simulink model "LabB_PIDOverRobot"  (R2020b)
settings: Solver=FixedStepDiscrete  StartTime=0.0  StopTime=inf  FixedStep=fSamplingPeriod  RelTol=1e-3  EnableMultiTasking=on
values from neighbouring files (symbols this model uses):
  acc_LSB_per_g = 16384    [GyroAccScaling.mat]
  acc_y_offset = 651.5    [OffsetData.mat]
  acc_z_offset = 170.75    [OffsetData.mat]
  fSamplingPeriod = 0.005    [LabB_ControllerOverSimulator_Discrete_Parameters.m]    (also in LabB_ControllerOverSimulator_Discrete_Parameters_conflict_copy_LAPTOP-FOGVCHE7_2020_11_15.m; LabB_ObserverAndControllerOverSimulator_Discrete_Parameters.m; LabC_6_3.m = 0.2; LabC_6_4.m = 0.067)
  fWheelRadius = 0.0216    [LoadRobotParameters.m]
  gyro_LSB_per_deg = 131    [GyroAccScaling.mat]
  gyro_x_offset = -193.125    [OffsetData.mat]
  iNumberOfEncoderSteps = 720    [LoadRobotParameters.m]
  kD = -0.87072    [LabB_ObserverAndControllerOverSimulator_Discrete_Parameters.m]    (also in LabB_ObserverOverSimulator_Continuous_Parameters.m; LabB_ObserverOverSimulator_Discrete_Parameters.m; LabC_6_6.m = 28.69)
  kI = -13776.6318    [LabB_ObserverAndControllerOverSimulator_Discrete_Parameters.m]    (also in LabB_ObserverOverSimulator_Continuous_Parameters.m; LabB_ObserverOverSimulator_Discrete_Parameters.m; LabC_6_6.m = 114.8)
  kP = -558.3481    [LabB_ObserverAndControllerOverSimulator_Discrete_Parameters.m]    (also in LabB_ObserverOverSimulator_Continuous_Parameters.m; LabB_ObserverOverSimulator_Discrete_Parameters.m; LabC_6_6.m = -9492)
undefined symbols (not defined in the file or in its folder): equ_offset
libraries: MinSegLibrary_M2V3 x3, simulink_extras x2, pid_lib x1, arduinolib x1
settings Model: FPTRunName=FPA_Reference  SimulationMode=external  ExtModeTrigDuration=2  Creator=Alec  LastModifiedBy=janes
settings DataIOCC: SaveFormat=Array  SaveOutput=off  SignalLogging=off  DSMLogging=off  SaveTime=off  ReturnWorkspaceOutputs=off
settings OptimizationCC: PassReuseOutputArgsThreshold=0  ExpressionDepthLimit=2147483647  MaxStackSize=64
settings DebuggingCC: UnderspecifiedInitializationDetection=Classic  MergeDetectMultiDrivingBlocksExec=none  ParameterTunabilityLossMsg=error  StateNameClashWarn=warning  SFUnexpectedBacktrackingDiag=warning  SFNoUnconditionalDefaultTransitionDiag=warning  SFExecutionAtInitializationDiag=none  ArithmeticOperatorsInVariantConditions=warning
settings HardwareCC: ProdBitPerInt=16  ProdBitPerPointer=16  ProdBitPerSizeT=16  ProdBitPerPtrDiffT=16  ProdLargestAtomicFloat=None  ProdWordSize=8  ProdHWDeviceType=Atmel->AVR  UseEmbeddedCoderFeatures=off
settings ModelReferenceCC: PropagateSignalLabelsOutOfModel=off
settings SFSimCC: SimUseLocalCustomCode=off  MATLABDynamicMemAlloc=off  CustomCodeUndefinedFunction=UseInterfaceOnly
settings RTWCC: Description=Embedded Coder  SystemTargetFile=ert.tlc  HardwareBoard=Arduino Mega 2560  TemplateMakefile=ert_default_tmf  GenerateReport=on  RTWVerbose=off  RTWUseLocalCustomCode=off  Toolchain=Arduino AVR  BuildConfiguration=Faster Runs  LaunchReport=on
settings CodeAppCC: ForceParamTrailComments=on  OperatorAnnotations=on  StateflowObjectComments=on  MATLABSourceComments=on
settings ERTTargetCC: ERTCustomFileBanners=off  SupportContinuousTime=on  SupportNonInlinedSFcns=on  RemoveResetFunc=off  SupportVariableSizeSignals=on  ModelStepFunctionPrototypeControlCompliant=off
settings ConfigComp: CovMetricSettings=dw  CovSaveCumulativeToWorkspaceVar=on  CovSaveSingleToWorkspaceVar=on  CovExternalEMLEnable=off

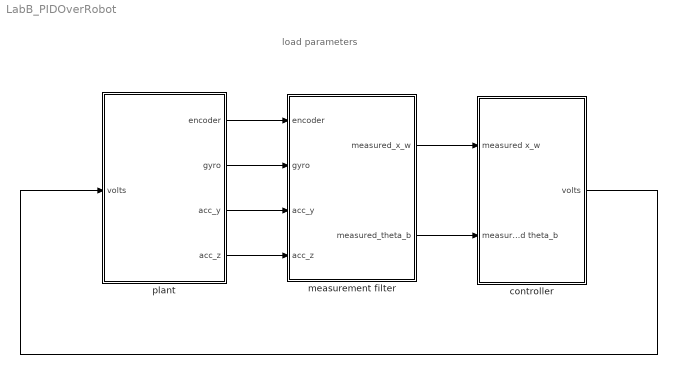
== system LabB_PIDOverRobot ==
  note: load parameters
  controller : Subsystem
  measurement filter : Subsystem
  plant : Subsystem
  wires:
  controller/1(volts) -> plant/1(volts)
  measurement filter/1(measured_x_w) -> controller/1(measured x_w)
  measurement filter/2(measured_theta_b) -> controller/2("measured theta_b ")
  plant/1(encoder) -> measurement filter/1(encoder)
  plant/2(gyro) -> measurement filter/2(gyro)
  plant/3(acc_y) -> measurement filter/3("acc_y ")
  plant/4(acc_z) -> measurement filter/4(acc_z)

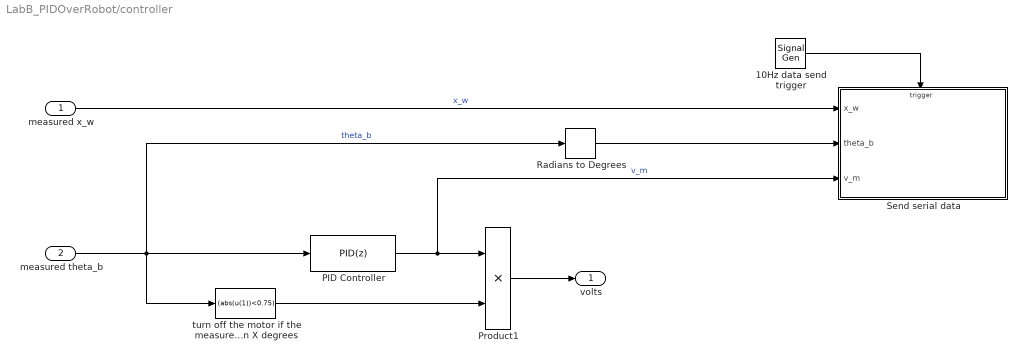
== system LabB_PIDOverRobot/controller ==
  measured x_w : Inport
  "measured theta_b " : Inport  Port=2
  10Hz data send trigger : SignalGenerator  WaveForm=sawtooth  Frequency=10
  PID Controller : pid_lib/PID Controller  Controller=PID  Form=Parallel  TimeDomain=Discrete-time  UseExternalTs=off  SampleTime=fSamplingPeriod  IntegratorMethod=Forward Euler  FilterMethod=Forward Euler  ControllerParametersSource=internal  P=kP  I=kI  D=kD  UseFilter=on  N=100  TunerSelectOption=Transfer Function Based (PID Tuner App)  InitialConditionSource=internal  InitialConditionForIntegrator=0  InitialConditionForFilter=0  DifferentiatorICPrevScaledInput=0  ExternalReset=none  TrackingMode=off  Kt=1  LimitOutput=on  SatLimitsSource=internal  UpperSaturationLimit=6  LowerSaturationLimit=-6  LinearizeAsGain=on  AntiWindupMode=back-calculation  Kb=1  POutMin=[]  POutMax=[]  IOutMin=[]  IOutMax=[]  DOutMin=[]  DOutMax=[]  NOutMin=[]  NOutMax=[]  SumOutMin=[]  SumOutMax=[]  SaturationOutMin=[]  SaturationOutMax=[]  PParamMin=[]  PParamMax=[]  IParamMin=[]  IParamMax=[]  DParamMin=[]  DParamMax=[]  NParamMin=[]  NParamMax=[]  KbParamMin=[]  KbParamMax=[]  KtParamMin=[]  KtParamMax=[]  KbOutMin=[]  KbOutMax=[]  KtOutMin=[]  KtOutMax=[]  IntegratorOutMin=[]  IntegratorOutMax=[]  FilterOutMin=[]  FilterOutMax=[]  SumI1OutMin=[]  SumI1OutMax=[]  SumI2OutMin=[]  SumI2OutMax=[]  SumI3OutMin=[]  SumI3OutMax=[]  SumI4OutMin=[]  SumI4OutMax=[]  SumDOutMin=[]  SumDOutMax=[]  DifferentiatorOutMin=[]  DifferentiatorOutMax=[]  FilterDiffOutCoefMin=[]  FilterDiffOutCoefMax=[]  ReciprocalOutMin=[]  ReciprocalOutMax=[]  SumDenOutMin=[]  SumDenOutMax=[]  SumNumOutMin=[]  SumNumOutMax=[]  DivideOutMin=[]  DivideOutMax=[]  UdiffTsProdOutMin=[]  UdiffTsProdOutMax=[]  NTsProdOutMin=[]  NTsProdOutMax=[]  UintegralTsProdOutMin=[]  UintegralTsProdOutMax=[]  UngainTsProdOutMin=[]  UngainTsProdOutMax=[]  IntegratorContinuousStateAttributes=''  IntegratorStateMustResolveToSignalObject=off  IntegratorRTWStateStorageClass=Auto  FilterContinuousStateAttributes=''  FilterStateMustResolveToSignalObject=off  FilterRTWStateStorageClass=Auto  ParallelPVariant=InternalParameters  IdealPVariant=Disabled  IVariant=InternalParameters  DVariant=InternalParameters  IntegratorVariant=Discrete  SatVariant=Enabled  AWVariant=BackCalculation  PCopyVariant=Disabled  TRVariant=Disabled  FdbkBlocksVariant=Forward  IdealPFdbkVariant=Disabled  SatFdbkVariant=Disabled  DerivativeFilterVariant=ForwardEulerFilter  NVariant=InternalParameters  NCopyVariant=Disabled  FilterICVariant=InternalICsFilter  IntegratorICVariant=InternalICs  ExternalResetVariant=Disabled  TRSumVariant=Passthrough  SumFdbkVariant=Disabled  SumVariant=Sum_PID  TsampFilterVariant=InternalTs  TsampNgainVariant=Passthrough  TsampIntegralVariant=Passthrough  ExternalSaturationOutDataTypeStr=Inherit: Same as second input
  Product1 : Product  RndMeth=Zero
  Radians to Degrees : simulink_extras/Transformations/Radians to Degrees
  Send serial data : Subsystem  TreatAsAtomicUnit=on
  turn off the motor if the measured angle is greater than X degrees : Fcn  Expr=(abs(u(1))<0.75)
  volts : Outport  VectorParamsAs1DForOutWhenUnconnected=off
  wires:
  "measured theta_b "/1 -> Radians to Degrees/1, turn off the motor if the measured angle is greater than X degrees/1, PID Controller/1  "theta_b"
  Product1/1 -> volts/1
  turn off the motor if the measured angle is greater than X degrees/1 -> Product1/2
  PID Controller/1 -> Send serial data/3(v_m), Product1/1  "v_m"
  10Hz data send trigger/1 -> Send serial data/Trigger
  measured x_w/1 -> Send serial data/1(x_w)  "x_w"
  Radians to Degrees/1 -> Send serial data/2(theta_b)

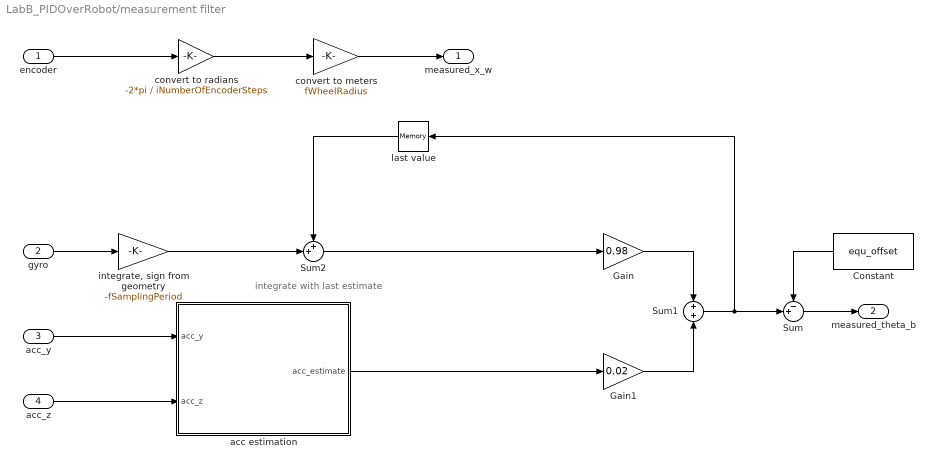
== system LabB_PIDOverRobot/measurement filter ==
  note: integrate with last estimate
  encoder : Inport
  gyro : Inport  Port=2
  "acc_y " : Inport  Port=3
  acc_z : Inport  Port=4
  Constant : Constant  Value=equ_offset
  Gain : Gain  Gain=0.98
  Gain1 : Gain  Gain=0.02
  Sum : Sum  Inputs=-+|
  Sum1 : Sum
  Sum2 : Sum  Inputs=++|
  acc estimation : Subsystem
  convert to radians : Gain  Gain=-2*pi / iNumberOfEncoderSteps  OutDataTypeStr=Inherit: Same as input
  convert to meters : Gain  Gain=fWheelRadius  OutDataTypeStr=Inherit: Same as input
  "integrate, sign from geometry" : Gain  Gain=-fSamplingPeriod
  last value : Memory
  measured_x_w : Outport  VectorParamsAs1DForOutWhenUnconnected=off
  measured_theta_b : Outport  Port=2  VectorParamsAs1DForOutWhenUnconnected=off
  wires:
  convert to radians/1 -> convert to meters/1
  encoder/1 -> convert to radians/1
  Sum1/1 -> Sum/2, last value/1
  convert to meters/1 -> measured_x_w/1
  "integrate, sign from geometry"/1 -> Sum2/2
  acc_z/1 -> acc estimation/2("acc_z ")
  Gain1/1 -> Sum1/2
  Sum2/1 -> Gain/1
  acc estimation/1(acc_estimate) -> Gain1/1
  Gain/1 -> Sum1/1
  gyro/1 -> "integrate, sign from geometry"/1
  last value/1 -> Sum2/1
  "acc_y "/1 -> acc estimation/1(acc_y)
  Sum/1 -> measured_theta_b/1
  Constant/1 -> Sum/1

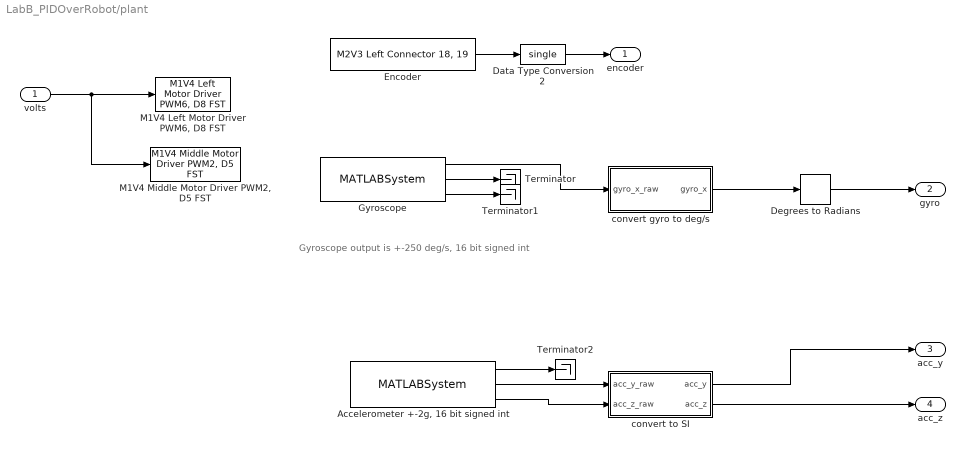
== system LabB_PIDOverRobot/plant ==
  note: Gyroscope output is +-250 deg/s, 16 bit signed int
  volts : Inport
  "Accelerometer +-2g, 16 bit signed int" : MATLABSystem  System=soMPU6050Accel  SimulateUsing=Code generation
      mask Type: soMPU6050Accel
      mask Display:
      | disp('soMPU6050Accel');
      | port_label('output',1,'xaccel');
      | port_label('output',2,'yaccel');
      | port_label('output',3,'zaccel');
  Data Type Conversion2 : DataTypeConversion  OutDataTypeStr=single
  Degrees to Radians : simulink_extras/Transformations/Degrees to Radians
  Encoder : MinSegLibrary_M2V3/M2V3 Left Connector 18, 19  Encoder=1  PinA=19  PinB=18
      settings: SourceProductName=Rensselaer Arduino Support Package
  Gyroscope : MATLABSystem  System=soMPU6050Gyro  DLPFmode=0
      mask Type: soMPU6050Gyro
      mask Display:
      | disp('soMPU6050Gyro');
      | port_label('output',1,'xvel');
      | port_label('output',2,'yvel');
      | port_label('output',3,'zvel');
  "M1V4 Left Motor Driver PWM6, D8 FST" : MinSegLibrary_M2V3/M1V4 Left Motor Driver PWM6, D8 FST  Vsupply=7.2
      settings: SourceProductName=Rensselaer Arduino Support Package
  "M1V4 Middle Motor Driver PWM2, D5 FST" : MinSegLibrary_M2V3/M1V4 Middle Motor Driver PWM2, D5 FST  Vsupply=7.2
      settings: SourceProductName=Rensselaer Arduino Support Package
  Terminator : Terminator
  Terminator1 : Terminator
  Terminator2 : Terminator
  convert gyro to deg/s : Subsystem
  convert to SI : Subsystem
  encoder : Outport  VectorParamsAs1DForOutWhenUnconnected=off
  gyro : Outport  Port=2  VectorParamsAs1DForOutWhenUnconnected=off
  acc_y : Outport  Port=3
  acc_z : Outport  Port=4
  wires:
  Encoder/1 -> Data Type Conversion2/1
  Data Type Conversion2/1 -> encoder/1
  volts/1 -> "M1V4 Middle Motor Driver PWM2, D5 FST"/1, "M1V4 Left Motor Driver PWM6, D8 FST"/1
  convert to SI/1(acc_y) -> acc_y/1
  "Accelerometer +-2g, 16 bit signed int"/2 -> convert to SI/1("acc_y_raw ")
  Gyroscope/3 -> Terminator1/1
  "Accelerometer +-2g, 16 bit signed int"/1 -> Terminator2/1
  Gyroscope/1 -> convert gyro to deg/s/1(gyro_x_raw)
  "Accelerometer +-2g, 16 bit signed int"/3 -> convert to SI/2(acc_z_raw)
  convert to SI/2(acc_z) -> acc_z/1
  convert gyro to deg/s/1(gyro_x) -> Degrees to Radians/1
  Degrees to Radians/1 -> gyro/1
  Gyroscope/2 -> Terminator/1

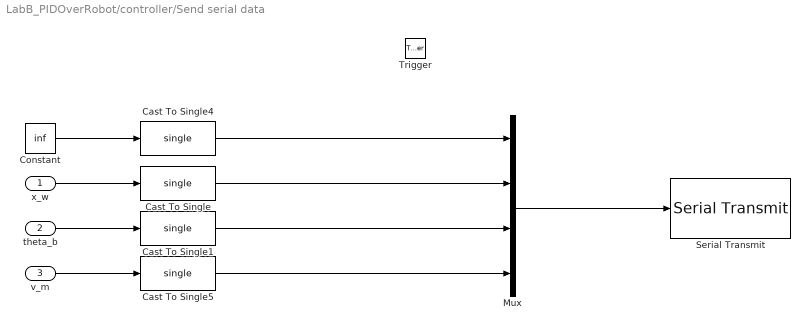
== system LabB_PIDOverRobot/controller/Send serial data ==
  x_w : Inport
  theta_b : Inport  Port=2
  v_m : Inport  Port=3
  Trigger : TriggerPort  TriggerType=falling  VariantControl=Variant
  Cast To Single{,1,4..5} (4 alike) : DataTypeConversion  OutDataTypeStr=single
  Constant : Constant  Value=inf  OutDataTypeStr=single
  Mux : Mux
  Serial Transmit : arduinolib/Serial Transmit  portNumber=0  sendmode=write  sendformat=Decimal  floatprecision=2  blockPlatform=arduino
  wires:
  Cast To Single1/1 -> Mux/3
  Cast To Single/1 -> Mux/2
  theta_b/1 -> Cast To Single1/1
  x_w/1 -> Cast To Single/1
  Constant/1 -> Cast To Single4/1
  v_m/1 -> Cast To Single5/1
  Cast To Single5/1 -> Mux/4
  Cast To Single4/1 -> Mux/1
  Mux/1 -> Serial Transmit/1

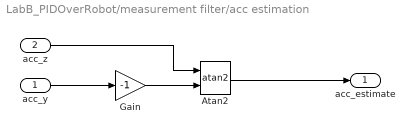
== system LabB_PIDOverRobot/measurement filter/acc estimation ==
  acc_y : Inport
  "acc_z " : Inport  Port=2
  Atan2 : Trigonometry  Operator=atan2
  Gain : Gain  Gain=-1
  acc_estimate : Outport  VectorParamsAs1DForOutWhenUnconnected=off
  wires:
  Gain/1 -> Atan2/2
  acc_y/1 -> Gain/1
  "acc_z "/1 -> Atan2/1
  Atan2/1 -> acc_estimate/1

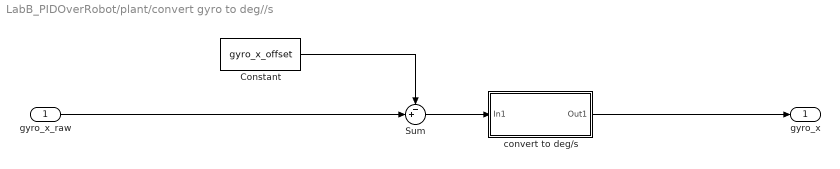
== system LabB_PIDOverRobot/plant/convert gyro to deg//s ==
  gyro_x_raw : Inport
  Constant : Constant  Value=gyro_x_offset
  Sum : Sum  Inputs=-+|
  convert to deg/s : Subsystem
  gyro_x : Outport  VectorParamsAs1DForOutWhenUnconnected=off
  wires:
  gyro_x_raw/1 -> Sum/2
  Sum/1 -> convert to deg/s/1(In1)
  convert to deg/s/1(Out1) -> gyro_x/1
  Constant/1 -> Sum/1

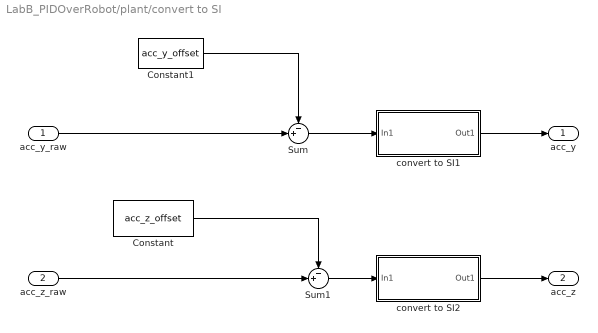
== system LabB_PIDOverRobot/plant/convert to SI ==
  "acc_y_raw " : Inport
  acc_z_raw : Inport  Port=2
  Constant : Constant  Value=acc_z_offset
  Constant1 : Constant  Value=acc_y_offset
  Sum : Sum  Inputs=-+|
  Sum1 : Sum  Inputs=-+|
  convert to SI1 : Subsystem
  convert to SI2 : Subsystem
  acc_y : Outport  VectorParamsAs1DForOutWhenUnconnected=off
  acc_z : Outport  Port=2  VectorParamsAs1DForOutWhenUnconnected=off
  wires:
  convert to SI1/1(Out1) -> acc_y/1
  convert to SI2/1(Out1) -> acc_z/1
  Sum/1 -> convert to SI1/1(In1)
  "acc_y_raw "/1 -> Sum/2
  Sum1/1 -> convert to SI2/1(In1)
  acc_z_raw/1 -> Sum1/2
  Constant/1 -> Sum1/1
  Constant1/1 -> Sum/1

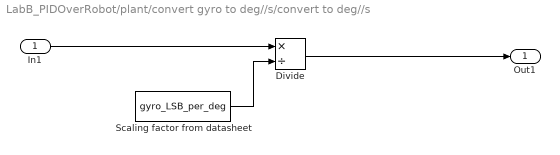
== system LabB_PIDOverRobot/plant/convert gyro to deg//s/convert to deg//s ==
  In1 : Inport
  Divide : Product  Inputs=*/
  Scaling factor from datasheet : Constant  Value=gyro_LSB_per_deg
  Out1 : Outport  VectorParamsAs1DForOutWhenUnconnected=off
  wires:
  Scaling factor from datasheet/1 -> Divide/2
  In1/1 -> Divide/1
  Divide/1 -> Out1/1

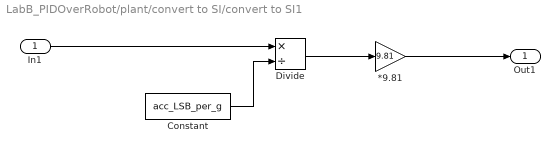
== system LabB_PIDOverRobot/plant/convert to SI/convert to SI1 ==
  In1 : Inport
  *9.81 : Gain  Gain=9.81
  Constant : Constant  Value=acc_LSB_per_g
  Divide : Product  Inputs=*/
  Out1 : Outport  VectorParamsAs1DForOutWhenUnconnected=off
  wires:
  Constant/1 -> Divide/2
  In1/1 -> Divide/1
  *9.81/1 -> Out1/1
  Divide/1 -> *9.81/1

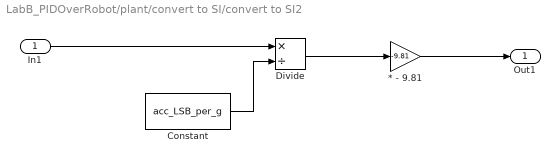
== system LabB_PIDOverRobot/plant/convert to SI/convert to SI2 ==
  In1 : Inport
  * - 9.81 : Gain  Gain=-9.81
  Constant : Constant  Value=acc_LSB_per_g
  Divide : Product  Inputs=*/
  Out1 : Outport  VectorParamsAs1DForOutWhenUnconnected=off
  wires:
  Constant/1 -> Divide/2
  In1/1 -> Divide/1
  * - 9.81/1 -> Out1/1
  Divide/1 -> * - 9.81/1
